simulink model "tank_reactor_no_error_dyn"  (R2020a)
settings: Solver=FixedStepAuto  StartTime=0.0  StopTime=options.T_train  FixedStep=options.dt  RelTol=1e-3
PreLoadFcn:
  | load PIDGainSchedExample.mat
model workspace (MAT data in the model file):
  op_snapshot1 : handle (value not decoded)
undefined symbols (not defined in the file or in its folder): C, Controllers, D, I, N, options, P, sigbuilder_block
libraries: neural x132, simulink x2, simulink_need_slupdate x1
(part 4 of 6)

== system tank_reactor_no_error_dyn/NN/Layer 3/Delays 1 ==
  "p{3}" : Inport  PortDimensions=30
      mask Display: e = 0.06;c1 = [120 230 180]/255;c2 = ([120 230 180]+0)/(256+128);c3 = ([120 230 180]+128)/(256+128);patch([0 1 1 0],[0 0 1 1],c1);patch([0 1 1 1-e 1-e 0+e],[0 0 1 1-e 0+e 0+e],c2);patch([0 0 1 1-e 0+e 0+e],[0 1 1 1-e 1-e 0+e],c3);plot([0 1 1 0 0],[0 0 1 1 0]);
  mux : Mux  Inputs=1
      mask Display: e = 0.06;c1 = [120 150 230]/255;c2 = ([120 150 230]+0)/383;c3 = ([120 150 230]+128)/383;patch([0 1 1 0],[0 0 1 1],c1);patch([0 1 1 1-e 1-e 0+e],[0 0 1 1-e 0+e 0+e],c2);patch([0 0 1 1-e 0+e 0+e],[0 1 1 1-e 1-e 0+e],c3);plot([0 1 1 0 0],[0 0 1 1 0]);disp('Mux')
  "pd{3,2}" : Outport
      mask Display: e = 0.06;c1 = [120 230 180]/255;c2 = ([120 230 180]+0)/(256+128);c3 = ([120 230 180]+128)/(256+128);patch([0 1 1 0],[0 0 1 1],c1);patch([0 1 1 1-e 1-e 0+e],[0 0 1 1-e 0+e 0+e],c2);patch([0 0 1 1-e 0+e 0+e],[0 1 1 1-e 1-e 0+e],c3);plot([0 1 1 0 0],[0 0 1 1 0]);
  wires:
  "p{3}"/1 -> mux/1
  mux/1 -> "pd{3,2}"/1

== system tank_reactor_no_error_dyn/NN/Layer 3/LW{3,2} ==
  "ad{3,2}" : Inport  PortDimensions=30
      mask Display: e = 0.06;c1 = [120 230 180]/255;c2 = ([120 230 180]+0)/(256+128);c3 = ([120 230 180]+128)/(256+128);patch([0 1 1 0],[0 0 1 1],c1);patch([0 1 1 1-e 1-e 0+e],[0 0 1 1-e 0+e 0+e],c2);patch([0 0 1 1-e 0+e 0+e],[0 1 1 1-e 1-e 0+e],c3);plot([0 1 1 0 0],[0 0 1 1 0]);
  "IW{3,2}(1,:)'" : Constant  Value=[-0.0511636272727241381286233945502317510545253753662109375;-0.228435345687879765019800970549113117158412933349609375;0.09378185793298553230012970516327186487615108489990234375;0.30732968004933403083356324714259244501590728759765625;-0.0026202039604571948812339332590681806323118507862091064453125;-0.1112622079165584698667856855536228977143764495849609375;-0.10130639427641263683455008504097349941730499267578125;0.06769739116965713121576442290461272932589054107666015625;-0.1255451148000425731776630300373653881251811981201171875;-0.07607780761738723585008159489007084630429744720458984375;-0.08226752934348340040582314713901723735034465789794921875;-0.01408145722205182519271016161610532435588538646697998046875;-0.02022664868012079286696547342216945253312587738037109375;-0.132883871763963157253130020762910135090351104736328125;-0.324757632621128611294381016705301590263843536376953125;-0.0153480898639730863053376452853626688010990619659423828125;0.01046282805957223123460853031474471208639442920684814453125;-0.00411317650747298861613199250086836400441825389862060546875;0.06722186949668589039941224427820998243987560272216796875;0.0896070865747360667530330147201311774551868438720703125;-0.254826262873892039895196148791001178324222564697265625;-0.02907748808419595432095405840300372801721096038818359375;0.1823688820218593298339015973397181369364261627197265625;-0.07852964486181500392003584920530556701123714447021484375;0.287449325203550654084239113217336125671863555908203125;-0.0266849151074926189963765210677593131549656391143798828125;0.041099048807482808920443773104125284589827060699462890625;0.081766120098062444743192145324428565800189971923828125;0.45293085224205065220104415857349522411823272705078125;-0.343650288483047849918960991999483667314052581787109375]
      mask Display: e = 0.06;c1 = [120 150 230]/255;c2 = ([120 150 230]+0)/383;c3 = ([120 150 230]+128)/383;patch([0 1 1 0],[0 0 1 1],c1);patch([0 1 1 1-e 1-e 0+e],[0 0 1 1-e 0+e 0+e],c2);patch([0 0 1 1-e 0+e 0+e],[0 1 1 1-e 1-e 0+e],c3);plot([0 1 1 0 0],[0 0 1 1 0]);disp('weights');
  Mux : Mux  Inputs=1
      mask Display: e = 0.06;c1 = [120 150 230]/255;c2 = ([120 150 230]+0)/383;c3 = ([120 150 230]+128)/383;patch([0 1 1 0],[0 0 1 1],c1);patch([0 1 1 1-e 1-e 0+e],[0 0 1 1-e 0+e 0+e],c2);patch([0 0 1 1-e 0+e 0+e],[0 1 1 1-e 1-e 0+e],c3);plot([0 1 1 0 0],[0 0 1 1 0]);disp('Mux');
  dotprod1 : neural/Weight Functions/dotprod
  "lz{3,2}" : Outport
      mask Display: e = 0.06;c1 = [120 230 180]/255;c2 = ([120 230 180]+0)/(256+128);c3 = ([120 230 180]+128)/(256+128);patch([0 1 1 0],[0 0 1 1],c1);patch([0 1 1 1-e 1-e 0+e],[0 0 1 1-e 0+e 0+e],c2);patch([0 0 1 1-e 0+e 0+e],[0 1 1 1-e 1-e 0+e],c3);plot([0 1 1 0 0],[0 0 1 1 0]);
  wires:
  "IW{3,2}(1,:)'"/1 -> dotprod1/1
  "ad{3,2}"/1 -> dotprod1/2
  dotprod1/1 -> Mux/1
  Mux/1 -> "lz{3,2}"/1

== system tank_reactor_no_error_dyn/NN_cex_1/Layer 1/Delays 1 ==
  "p{1}" : Inport  PortDimensions=8
      mask Display: e = 0.06;c1 = [120 230 180]/255;c2 = ([120 230 180]+0)/(256+128);c3 = ([120 230 180]+128)/(256+128);patch([0 1 1 0],[0 0 1 1],c1);patch([0 1 1 1-e 1-e 0+e],[0 0 1 1-e 0+e 0+e],c2);patch([0 0 1 1-e 0+e 0+e],[0 1 1 1-e 1-e 0+e],c3);plot([0 1 1 0 0],[0 0 1 1 0]);
  mux : Mux  Inputs=1
      mask Display: e = 0.06;c1 = [120 150 230]/255;c2 = ([120 150 230]+0)/383;c3 = ([120 150 230]+128)/383;patch([0 1 1 0],[0 0 1 1],c1);patch([0 1 1 1-e 1-e 0+e],[0 0 1 1-e 0+e 0+e],c2);patch([0 0 1 1-e 0+e 0+e],[0 1 1 1-e 1-e 0+e],c3);plot([0 1 1 0 0],[0 0 1 1 0]);disp('Mux')
  "pd{1,1}" : Outport
      mask Display: e = 0.06;c1 = [120 230 180]/255;c2 = ([120 230 180]+0)/(256+128);c3 = ([120 230 180]+128)/(256+128);patch([0 1 1 0],[0 0 1 1],c1);patch([0 1 1 1-e 1-e 0+e],[0 0 1 1-e 0+e 0+e],c2);patch([0 0 1 1-e 0+e 0+e],[0 1 1 1-e 1-e 0+e],c3);plot([0 1 1 0 0],[0 0 1 1 0]);
  wires:
  "p{1}"/1 -> mux/1
  mux/1 -> "pd{1,1}"/1

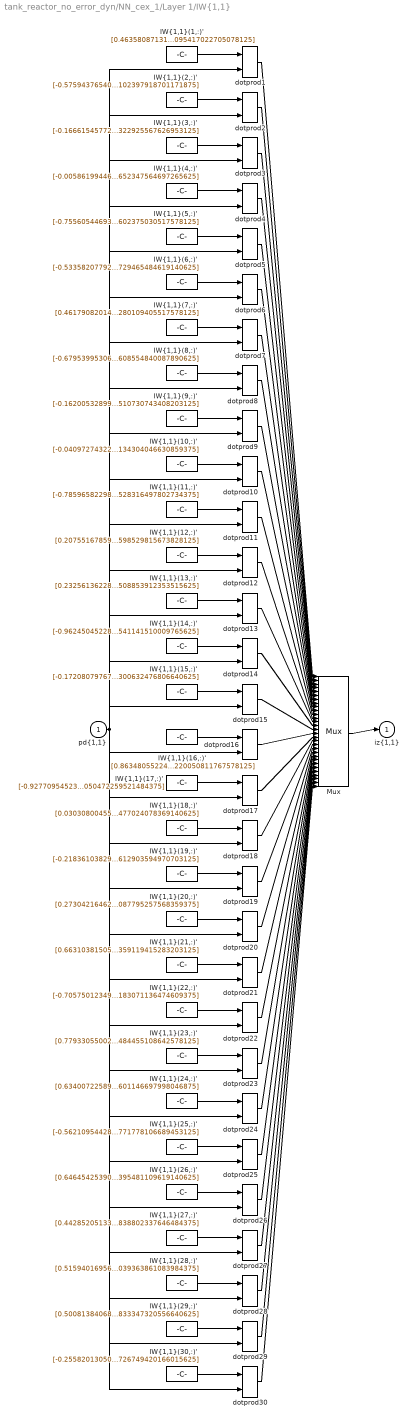
== system tank_reactor_no_error_dyn/NN_cex_1/Layer 1/IW{1,1} ==
  "pd{1,1}" : Inport  PortDimensions=8
      mask Display: e = 0.06;c1 = [120 230 180]/255;c2 = ([120 230 180]+0)/(256+128);c3 = ([120 230 180]+128)/(256+128);patch([0 1 1 0],[0 0 1 1],c1);patch([0 1 1 1-e 1-e 0+e],[0 0 1 1-e 0+e 0+e],c2);patch([0 0 1 1-e 0+e 0+e],[0 1 1 1-e 1-e 0+e],c3);plot([0 1 1 0 0],[0 0 1 1 0]);
  "IW{1,1}(1,:)'" : Constant  Value=[0.463580871318489851073962881855550222098827362060546875;-0.7904587112242886792756735303555615246295928955078125;0.57442801713559255016861015974427573382854461669921875;1.4978647593431768658689406947814859449863433837890625;-0.95724167897599621301907291126553900539875030517578125;0.064253678467424413245367986746714450418949127197265625;0.2444816783607909604913999146447167731821537017822265625;-0.2330448826646716320443175618493114598095417022705078125]
      mask Display: e = 0.06;c1 = [120 150 230]/255;c2 = ([120 150 230]+0)/383;c3 = ([120 150 230]+128)/383;patch([0 1 1 0],[0 0 1 1],c1);patch([0 1 1 1-e 1-e 0+e],[0 0 1 1-e 0+e 0+e],c2);patch([0 0 1 1-e 0+e 0+e],[0 1 1 1-e 1-e 0+e],c3);plot([0 1 1 0 0],[0 0 1 1 0]);disp('Weights');
  "IW{1,1}(10,:)'" : Constant  Value=[-0.040972743222529188489300366882162052206695079803466796875;1.3653833096036469552103653768426738679409027099609375;-0.91960544872284799566841684281826019287109375;-0.67287265316171274154299908332177437841892242431640625;-0.14617210117683787640174841726548038423061370849609375;0.380836409839925504883240137132816016674041748046875;0.0876222293789833683863577107331366278231143951416015625;1.256903587889906415142604600987397134304046630859375]
      mask Display: e = 0.06;c1 = [120 150 230]/255;c2 = ([120 150 230]+0)/383;c3 = ([120 150 230]+128)/383;patch([0 1 1 0],[0 0 1 1],c1);patch([0 1 1 1-e 1-e 0+e],[0 0 1 1-e 0+e 0+e],c2);patch([0 0 1 1-e 0+e 0+e],[0 1 1 1-e 1-e 0+e],c3);plot([0 1 1 0 0],[0 0 1 1 0]);disp('Weights');
  "IW{1,1}(11,:)'" : Constant  Value=[-0.7859658229803023754556079438771121203899383544921875;-0.52967905565982198456964624710963107645511627197265625;0.90365927008908764062056206967099569737911224365234375;-0.427517699502745929240887790001579560339450836181640625;-0.85982789438278517391012201187550090253353118896484375;-1.1238235294587177737213323780451901257038116455078125;-0.325401621469426693966653374445741064846515655517578125;-0.08553663223588357789051173085681512020528316497802734375]
      mask Display: e = 0.06;c1 = [120 150 230]/255;c2 = ([120 150 230]+0)/383;c3 = ([120 150 230]+128)/383;patch([0 1 1 0],[0 0 1 1],c1);patch([0 1 1 1-e 1-e 0+e],[0 0 1 1-e 0+e 0+e],c2);patch([0 0 1 1-e 0+e 0+e],[0 1 1 1-e 1-e 0+e],c3);plot([0 1 1 0 0],[0 0 1 1 0]);disp('Weights');
  "IW{1,1}(12,:)'" : Constant  Value=[0.2075516785995884794235877279788837768137454986572265625;-1.2880702182765999541658175076008774340152740478515625;0.55049483529810461224229811705299653112888336181640625;-0.3942878107891996108946841559372842311859130859375;0.78421997391049125258888352618669159710407257080078125;-0.0082326501651055657149402833283602376468479633331298828125;0.08183215105199100058985806072087143547832965850830078125;1.60118606217460968110799512942321598529815673828125]
      mask Display: e = 0.06;c1 = [120 150 230]/255;c2 = ([120 150 230]+0)/383;c3 = ([120 150 230]+128)/383;patch([0 1 1 0],[0 0 1 1],c1);patch([0 1 1 1-e 1-e 0+e],[0 0 1 1-e 0+e 0+e],c2);patch([0 0 1 1-e 0+e 0+e],[0 1 1 1-e 1-e 0+e],c3);plot([0 1 1 0 0],[0 0 1 1 0]);disp('Weights');
  "IW{1,1}(13,:)'" : Constant  Value=[0.2325613622819835690780365666796569712460041046142578125;0.6884494995406864603637586697004735469818115234375;0.91152589192887567559608896772260777652263641357421875;-0.974281841732740350181529720430262386798858642578125;0.561050562518456530369803658686578273773193359375;-0.36138030563152911955882018446573056280612945556640625;0.031805128071507038356457996997050940990447998046875;1.3856379731621599749047391014755703508853912353515625]
      mask Display: e = 0.06;c1 = [120 150 230]/255;c2 = ([120 150 230]+0)/383;c3 = ([120 150 230]+128)/383;patch([0 1 1 0],[0 0 1 1],c1);patch([0 1 1 1-e 1-e 0+e],[0 0 1 1-e 0+e 0+e],c2);patch([0 0 1 1-e 0+e 0+e],[0 1 1 1-e 1-e 0+e],c3);plot([0 1 1 0 0],[0 0 1 1 0]);disp('Weights');
  "IW{1,1}(14,:)'" : Constant  Value=[-0.96245045228366199463465591179556213319301605224609375;-1.2333069155908173986091469487291760742664337158203125;0.79278077813697100939549500253633596003055572509765625;0.6794397573296786507768274532281793653964996337890625;-0.527000734411264826206888756132684648036956787109375;0.787959872679240280746171265491284430027008056640625;-0.61877659409885932273454045571270398795604705810546875;-0.74362758890356295271573117133812047541141510009765625]
      mask Display: e = 0.06;c1 = [120 150 230]/255;c2 = ([120 150 230]+0)/383;c3 = ([120 150 230]+128)/383;patch([0 1 1 0],[0 0 1 1],c1);patch([0 1 1 1-e 1-e 0+e],[0 0 1 1-e 0+e 0+e],c2);patch([0 0 1 1-e 0+e 0+e],[0 1 1 1-e 1-e 0+e],c3);plot([0 1 1 0 0],[0 0 1 1 0]);disp('Weights');
  "IW{1,1}(15,:)'" : Constant  Value=[-0.1720807976720290788374967405616189353168010711669921875;1.6346800282565066009254906020942144095897674560546875;-1.5275045226209156279395529054454527795314788818359375;0.48163706898306113401986294775269925594329833984375;-1.4090195244134176011385761739802546799182891845703125;1.0074444406116940253781422143219970166683197021484375;0.149048248710748676426618430923554114997386932373046875;0.583897769695257640165664270170964300632476806640625]
      mask Display: e = 0.06;c1 = [120 150 230]/255;c2 = ([120 150 230]+0)/383;c3 = ([120 150 230]+128)/383;patch([0 1 1 0],[0 0 1 1],c1);patch([0 1 1 1-e 1-e 0+e],[0 0 1 1-e 0+e 0+e],c2);patch([0 0 1 1-e 0+e 0+e],[0 1 1 1-e 1-e 0+e],c3);plot([0 1 1 0 0],[0 0 1 1 0]);disp('Weights');
  "IW{1,1}(16,:)'" : Constant  Value=[0.8634805522466171279205582322902046144008636474609375;-0.826832306692147245286150791798718273639678955078125;-0.459024428825649588592483496540808118879795074462890625;-0.225724673917949036905383763951249420642852783203125;0.7769046624413535884201564840623177587985992431640625;0.07897558014084467281623602730178390629589557647705078125;-0.80444668751484471602708481441368348896503448486328125;-0.68029164592008506406983769920771010220050811767578125]
      mask Display: e = 0.06;c1 = [120 150 230]/255;c2 = ([120 150 230]+0)/383;c3 = ([120 150 230]+128)/383;patch([0 1 1 0],[0 0 1 1],c1);patch([0 1 1 1-e 1-e 0+e],[0 0 1 1-e 0+e 0+e],c2);patch([0 0 1 1-e 0+e 0+e],[0 1 1 1-e 1-e 0+e],c3);plot([0 1 1 0 0],[0 0 1 1 0]);disp('Weights');
  "IW{1,1}(17,:)'" : Constant  Value=[-0.92770954523786175460742242648848332464694976806640625;-0.70379974998822880660753753545577637851238250732421875;0.49312602053411913605174277108744718134403228759765625;0.2053519305894300484016667951436829753220081329345703125;0.81354542032451415689564555577817372977733612060546875;0.06332053666104490996513476375184836797416210174560546875;0.392478721046141398876017092334222979843616485595703125;0.9425610515299085445661830817698501050472259521484375]
      mask Display: e = 0.06;c1 = [120 150 230]/255;c2 = ([120 150 230]+0)/383;c3 = ([120 150 230]+128)/383;patch([0 1 1 0],[0 0 1 1],c1);patch([0 1 1 1-e 1-e 0+e],[0 0 1 1-e 0+e 0+e],c2);patch([0 0 1 1-e 0+e 0+e],[0 1 1 1-e 1-e 0+e],c3);plot([0 1 1 0 0],[0 0 1 1 0]);disp('Weights');
  "IW{1,1}(18,:)'" : Constant  Value=[0.030308004556539668017389743681633262895047664642333984375;0.72396828867836060528162533955764956772327423095703125;0.59124165685490748245456416043452918529510498046875;0.68453876641339650443995878958958201110363006591796875;0.873486939293690145547088832245208323001861572265625;-0.55859954329883254597888253556448034942150115966796875;0.88615609615319101965980053137172944843769073486328125;0.8792828693653904625904260683455504477024078369140625]
      mask Display: e = 0.06;c1 = [120 150 230]/255;c2 = ([120 150 230]+0)/383;c3 = ([120 150 230]+128)/383;patch([0 1 1 0],[0 0 1 1],c1);patch([0 1 1 1-e 1-e 0+e],[0 0 1 1-e 0+e 0+e],c2);patch([0 0 1 1-e 0+e 0+e],[0 1 1 1-e 1-e 0+e],c3);plot([0 1 1 0 0],[0 0 1 1 0]);disp('Weights');
  "IW{1,1}(19,:)'" : Constant  Value=[-0.21836103829253905583840378312743268907070159912109375;-1.7653401894298923480164376087486743927001953125;0.1304230755661318907900891872486681677401065826416015625;0.491037568941755153684169954431126825511455535888671875;0.880852994496023722348354567657224833965301513671875;0.4235760813815658831771315817604772746562957763671875;0.66282600456369278330015504252514801919460296630859375;-0.9759379388789650722202395627391524612903594970703125]
      mask Display: e = 0.06;c1 = [120 150 230]/255;c2 = ([120 150 230]+0)/383;c3 = ([120 150 230]+128)/383;patch([0 1 1 0],[0 0 1 1],c1);patch([0 1 1 1-e 1-e 0+e],[0 0 1 1-e 0+e 0+e],c2);patch([0 0 1 1-e 0+e 0+e],[0 1 1 1-e 1-e 0+e],c3);plot([0 1 1 0 0],[0 0 1 1 0]);disp('Weights');
  "IW{1,1}(2,:)'" : Constant  Value=[-0.57594376540703728917236503548338077962398529052734375;0.3962711625510093593760529984137974679470062255859375;-0.136957085468368655600812644479447044432163238525390625;0.90856087701288401614618805979262106120586395263671875;0.79920507598837442486683357856236398220062255859375;0.34068887162910421739780986172263510525226593017578125;0.94500832838045678574445673802983947098255157470703125;0.898124703405627666796817720751278102397918701171875]
      mask Display: e = 0.06;c1 = [120 150 230]/255;c2 = ([120 150 230]+0)/383;c3 = ([120 150 230]+128)/383;patch([0 1 1 0],[0 0 1 1],c1);patch([0 1 1 1-e 1-e 0+e],[0 0 1 1-e 0+e 0+e],c2);patch([0 0 1 1-e 0+e 0+e],[0 1 1 1-e 1-e 0+e],c3);plot([0 1 1 0 0],[0 0 1 1 0]);disp('Weights');
  "IW{1,1}(20,:)'" : Constant  Value=[0.27304216462729680170440360598149709403514862060546875;-1.2509692414445792163490978055051527917385101318359375;-0.59360848828293211187911992965382523834705352783203125;0.368084973461381192993968625160050578415393829345703125;-0.69093934225117104030999826136394403874874114990234375;0.52517178272850462139587079946068115532398223876953125;0.404032973990806620889770783833228051662445068359375;1.331038799733446520434654303244315087795257568359375]
      mask Display: e = 0.06;c1 = [120 150 230]/255;c2 = ([120 150 230]+0)/383;c3 = ([120 150 230]+128)/383;patch([0 1 1 0],[0 0 1 1],c1);patch([0 1 1 1-e 1-e 0+e],[0 0 1 1-e 0+e 0+e],c2);patch([0 0 1 1-e 0+e 0+e],[0 1 1 1-e 1-e 0+e],c3);plot([0 1 1 0 0],[0 0 1 1 0]);disp('Weights');
  "IW{1,1}(21,:)'" : Constant  Value=[0.66310381505613558150713515715324319899082183837890625;-0.5068485717960167225015766234719194471836090087890625;0.12251030924586096826356396150004002265632152557373046875;-0.453308562938941894682187694343156181275844573974609375;-1.4355076890545730439185945215285755693912506103515625;0.3534278437696298791337312650284729897975921630859375;-0.5361448701653539483658050812664441764354705810546875;-1.144453668082821451434938353486359119415283203125]
      mask Display: e = 0.06;c1 = [120 150 230]/255;c2 = ([120 150 230]+0)/383;c3 = ([120 150 230]+128)/383;patch([0 1 1 0],[0 0 1 1],c1);patch([0 1 1 1-e 1-e 0+e],[0 0 1 1-e 0+e 0+e],c2);patch([0 0 1 1-e 0+e 0+e],[0 1 1 1-e 1-e 0+e],c3);plot([0 1 1 0 0],[0 0 1 1 0]);disp('Weights');
  "IW{1,1}(22,:)'" : Constant  Value=[-0.7057501234978935666930510706151835620403289794921875;1.0777498783723895581232454787823371589183807373046875;0.9181709250255909449123237209278158843517303466796875;0.562010005880240637310407691984437406063079833984375;0.19714460918516607534911599941551685333251953125;1.147996642267212319410418785992078483104705810546875;-0.379426862334607761795268743298947811126708984375;-0.2291945269754227521019629421061836183071136474609375]
      mask Display: e = 0.06;c1 = [120 150 230]/255;c2 = ([120 150 230]+0)/383;c3 = ([120 150 230]+128)/383;patch([0 1 1 0],[0 0 1 1],c1);patch([0 1 1 1-e 1-e 0+e],[0 0 1 1-e 0+e 0+e],c2);patch([0 0 1 1-e 0+e 0+e],[0 1 1 1-e 1-e 0+e],c3);plot([0 1 1 0 0],[0 0 1 1 0]);disp('Weights');
  "IW{1,1}(23,:)'" : Constant  Value=[0.7793305500246863193325452812132425606250762939453125;-1.3963545070225931166163491070619784295558929443359375;-0.0197291050812327221908315522114207851700484752655029296875;0.6738974988460924020472475604037754237651824951171875;0.518831908117893814136323271668516099452972412109375;0.2877058771797831315808480212581343948841094970703125;-0.338558398751864164655245303947594948112964630126953125;-1.0022153826101807272408450444345362484455108642578125]
      mask Display: e = 0.06;c1 = [120 150 230]/255;c2 = ([120 150 230]+0)/383;c3 = ([120 150 230]+128)/383;patch([0 1 1 0],[0 0 1 1],c1);patch([0 1 1 1-e 1-e 0+e],[0 0 1 1-e 0+e 0+e],c2);patch([0 0 1 1-e 0+e 0+e],[0 1 1 1-e 1-e 0+e],c3);plot([0 1 1 0 0],[0 0 1 1 0]);disp('Weights');
  "IW{1,1}(24,:)'" : Constant  Value=[0.6340072258966429341597859092871658504009246826171875;0.37790605979201341568796124192886054515838623046875;-0.85645656739814957081335933253285475075244903564453125;-0.307011093371232057780417790127103216946125030517578125;0.3271156209610583953661944178747944533824920654296875;-0.05214857299869594953189988473241101019084453582763671875;1.3630762535353053710451831648242659866809844970703125;-1.1632957683929685543944287928752601146697998046875]
      mask Display: e = 0.06;c1 = [120 150 230]/255;c2 = ([120 150 230]+0)/383;c3 = ([120 150 230]+128)/383;patch([0 1 1 0],[0 0 1 1],c1);patch([0 1 1 1-e 1-e 0+e],[0 0 1 1-e 0+e 0+e],c2);patch([0 0 1 1-e 0+e 0+e],[0 1 1 1-e 1-e 0+e],c3);plot([0 1 1 0 0],[0 0 1 1 0]);disp('Weights');
  "IW{1,1}(25,:)'" : Constant  Value=[-0.56210954428920822945059398989542387425899505615234375;-0.36545828277500336245253720335313118994235992431640625;1.0061415530919173288992851666989736258983612060546875;-0.75339005875760989283662638626992702484130859375;0.80492991378725620155165643154759891331195831298828125;-0.01355985355531138907003718685473359073512256145477294921875;-0.449973166387047929237752441622433252632617950439453125;1.13479554730583931387855045613832771778106689453125]
      mask Display: e = 0.06;c1 = [120 150 230]/255;c2 = ([120 150 230]+0)/383;c3 = ([120 150 230]+128)/383;patch([0 1 1 0],[0 0 1 1],c1);patch([0 1 1 1-e 1-e 0+e],[0 0 1 1-e 0+e 0+e],c2);patch([0 0 1 1-e 0+e 0+e],[0 1 1 1-e 1-e 0+e],c3);plot([0 1 1 0 0],[0 0 1 1 0]);disp('Weights');
  "IW{1,1}(26,:)'" : Constant  Value=[0.64645425390136879162383820585091598331928253173828125;0.5379115281036155327143433169112540781497955322265625;0.98482449266796734388407230653683654963970184326171875;-1.234152891743236946098249973147176206111907958984375;0.552845338795752372362812820938415825366973876953125;-0.74973727573836124182804496740573085844516754150390625;-0.39753604357000338342942313829553313553333282470703125;0.37774497687728614270241678241291083395481109619140625]
      mask Display: e = 0.06;c1 = [120 150 230]/255;c2 = ([120 150 230]+0)/383;c3 = ([120 150 230]+128)/383;patch([0 1 1 0],[0 0 1 1],c1);patch([0 1 1 1-e 1-e 0+e],[0 0 1 1-e 0+e 0+e],c2);patch([0 0 1 1-e 0+e 0+e],[0 1 1 1-e 1-e 0+e],c3);plot([0 1 1 0 0],[0 0 1 1 0]);disp('Weights');
  "IW{1,1}(27,:)'" : Constant  Value=[0.442852051339611085811753810048685409128665924072265625;-0.1612759616178441046674407743921619839966297149658203125;-1.059514801227666946914496293175034224987030029296875;-0.31801079923491604173335645100451074540615081787109375;1.31667604694982731672325826366432011127471923828125;-0.196637959511739401907703950200811959803104400634765625;-0.84257433986396723657463780909893102943897247314453125;-0.73562573460771873978814028305350802838802337646484375]
      mask Display: e = 0.06;c1 = [120 150 230]/255;c2 = ([120 150 230]+0)/383;c3 = ([120 150 230]+128)/383;patch([0 1 1 0],[0 0 1 1],c1);patch([0 1 1 1-e 1-e 0+e],[0 0 1 1-e 0+e 0+e],c2);patch([0 0 1 1-e 0+e 0+e],[0 1 1 1-e 1-e 0+e],c3);plot([0 1 1 0 0],[0 0 1 1 0]);disp('Weights');
  "IW{1,1}(28,:)'" : Constant  Value=[0.515940169569911066815848244004882872104644775390625;0.326390302099289819626193320800666697323322296142578125;0.79363286471308303049454480060376226902008056640625;0.53611866584574408012286994562600739300251007080078125;-0.87791311431382024199621127991122193634510040283203125;-0.1311120155577295831594852870694012381136417388916015625;1.1060321036358544688482652418315410614013671875;-0.81245786194538227587003120788722299039363861083984375]
      mask Display: e = 0.06;c1 = [120 150 230]/255;c2 = ([120 150 230]+0)/383;c3 = ([120 150 230]+128)/383;patch([0 1 1 0],[0 0 1 1],c1);patch([0 1 1 1-e 1-e 0+e],[0 0 1 1-e 0+e 0+e],c2);patch([0 0 1 1-e 0+e 0+e],[0 1 1 1-e 1-e 0+e],c3);plot([0 1 1 0 0],[0 0 1 1 0]);disp('Weights');
  "IW{1,1}(29,:)'" : Constant  Value=[0.50081384068591983105278586663189344108104705810546875;0.70784116501752458727736438959254883229732513427734375;-0.54083562909659033124398774816654622554779052734375;-0.4016607451257583338843915043980814516544342041015625;-0.637187205003586942808624371537007391452789306640625;-1.3621243366178481526418408975587226450443267822265625;1.1372953341399416604673433539574034512042999267578125;-0.7814124788651357622626392185338772833347320556640625]
      mask Display: e = 0.06;c1 = [120 150 230]/255;c2 = ([120 150 230]+0)/383;c3 = ([120 150 230]+128)/383;patch([0 1 1 0],[0 0 1 1],c1);patch([0 1 1 1-e 1-e 0+e],[0 0 1 1-e 0+e 0+e],c2);patch([0 0 1 1-e 0+e 0+e],[0 1 1 1-e 1-e 0+e],c3);plot([0 1 1 0 0],[0 0 1 1 0]);disp('Weights');
  "IW{1,1}(3,:)'" : Constant  Value=[-0.1666154577238947442907601725892163813114166259765625;-0.6536488119383376815818564864457584917545318603515625;-1.0562606311580997608956522526568733155727386474609375;1.135074772634802275916854341630823910236358642578125;0.631701996163486878543835700838826596736907958984375;-1.0490198465701379149095373577438294887542724609375;-0.281305602571892687802090904369833879172801971435546875;-0.2419406811468441109713722880769637413322925567626953125]
      mask Display: e = 0.06;c1 = [120 150 230]/255;c2 = ([120 150 230]+0)/383;c3 = ([120 150 230]+128)/383;patch([0 1 1 0],[0 0 1 1],c1);patch([0 1 1 1-e 1-e 0+e],[0 0 1 1-e 0+e 0+e],c2);patch([0 0 1 1-e 0+e 0+e],[0 1 1 1-e 1-e 0+e],c3);plot([0 1 1 0 0],[0 0 1 1 0]);disp('Weights');
  "IW{1,1}(30,:)'" : Constant  Value=[-0.255820130507038723255419654378783889114856719970703125;-0.42046638486646104038158000548719428479671478271484375;0.94480030775071865978276264286250807344913482666015625;1.46246777067761968282866291701793670654296875;-0.94321670011016112145085799056687392294406890869140625;-0.131027866533403980486838236174662597477436065673828125;0.97966607272397465688840156872174702584743499755859375;-0.414381316283911671494166739648790098726749420166015625]
      mask Display: e = 0.06;c1 = [120 150 230]/255;c2 = ([120 150 230]+0)/383;c3 = ([120 150 230]+128)/383;patch([0 1 1 0],[0 0 1 1],c1);patch([0 1 1 1-e 1-e 0+e],[0 0 1 1-e 0+e 0+e],c2);patch([0 0 1 1-e 0+e 0+e],[0 1 1 1-e 1-e 0+e],c3);plot([0 1 1 0 0],[0 0 1 1 0]);disp('Weights');
  "IW{1,1}(4,:)'" : Constant  Value=[-0.005861994462960277464669278657538598054088652133941650390625;0.310384610035220942503286778446636162698268890380859375;-0.303985715566599645764966908245696686208248138427734375;1.532457273094987026951230291160754859447479248046875;0.14221060335721869005709550037863664329051971435546875;-0.2424428009628119828899883714257157407701015472412109375;0.78518710237456657008436877731583081185817718505859375;1.1900275375553894807723054327652789652347564697265625]
      mask Display: e = 0.06;c1 = [120 150 230]/255;c2 = ([120 150 230]+0)/383;c3 = ([120 150 230]+128)/383;patch([0 1 1 0],[0 0 1 1],c1);patch([0 1 1 1-e 1-e 0+e],[0 0 1 1-e 0+e 0+e],c2);patch([0 0 1 1-e 0+e 0+e],[0 1 1 1-e 1-e 0+e],c3);plot([0 1 1 0 0],[0 0 1 1 0]);disp('Weights');
  "IW{1,1}(5,:)'" : Constant  Value=[-0.7556054469320427902090386851341463625431060791015625;-1.1675269259961778001155607853434048593044281005859375;0.357343037332967627950353062260546721518039703369140625;-1.2615101675971087669125836328021250665187835693359375;0.318800595041070999879906366913928650319576263427734375;0.11144197081600955290259236107885953970253467559814453125;0.331933459356202720247352999649592675268650054931640625;0.1749402223806457989940810193729703314602375030517578125]
      mask Display: e = 0.06;c1 = [120 150 230]/255;c2 = ([120 150 230]+0)/383;c3 = ([120 150 230]+128)/383;patch([0 1 1 0],[0 0 1 1],c1);patch([0 1 1 1-e 1-e 0+e],[0 0 1 1-e 0+e 0+e],c2);patch([0 0 1 1-e 0+e 0+e],[0 1 1 1-e 1-e 0+e],c3);plot([0 1 1 0 0],[0 0 1 1 0]);disp('Weights');
  "IW{1,1}(6,:)'" : Constant  Value=[-0.533582077924919406797243937035091221332550048828125;-0.1769956811210130764866477193208993412554264068603515625;-0.68676284949857790973481996843474917113780975341796875;-0.2768405634972224138579122154624201357364654541015625;-0.85842097286933805033726230249158106744289398193359375;0.317723199909580367172878823112114332616329193115234375;-1.10436479719843827496106314356438815593719482421875;0.8243658839545775496304713669815100729465484619140625]
      mask Display: e = 0.06;c1 = [120 150 230]/255;c2 = ([120 150 230]+0)/383;c3 = ([120 150 230]+128)/383;patch([0 1 1 0],[0 0 1 1],c1);patch([0 1 1 1-e 1-e 0+e],[0 0 1 1-e 0+e 0+e],c2);patch([0 0 1 1-e 0+e 0+e],[0 1 1 1-e 1-e 0+e],c3);plot([0 1 1 0 0],[0 0 1 1 0]);disp('Weights');
  "IW{1,1}(7,:)'" : Constant  Value=[0.461790820143882341231034160955459810793399810791015625;0.9523723514546293955618239124305546283721923828125;-0.86591776759901872839719771945965476334095001220703125;0.2034614325072331142418846638975082896649837493896484375;-1.0535322448098103365055067115463316440582275390625;0.96893238416265947687833204327034763991832733154296875;0.5560285087582921281779135824763216078281402587890625;-0.73762414930330699736060751092736609280109405517578125]
      mask Display: e = 0.06;c1 = [120 150 230]/255;c2 = ([120 150 230]+0)/383;c3 = ([120 150 230]+128)/383;patch([0 1 1 0],[0 0 1 1],c1);patch([0 1 1 1-e 1-e 0+e],[0 0 1 1-e 0+e 0+e],c2);patch([0 0 1 1-e 0+e 0+e],[0 1 1 1-e 1-e 0+e],c3);plot([0 1 1 0 0],[0 0 1 1 0]);disp('Weights');
  "IW{1,1}(8,:)'" : Constant  Value=[-0.679539953065417368094358607777394354343414306640625;-0.675914190639570033880545452120713889598846435546875;-0.97077223646583943317267539896420203149318695068359375;-0.08346642929951418599099355333237326703965663909912109375;-0.98150656874792618911129693515249527990818023681640625;0.732775463199345278297869299422018229961395263671875;0.89468062331483999560788333837990649044513702392578125;-0.57336653345065580200667909593903459608554840087890625]
      mask Display: e = 0.06;c1 = [120 150 230]/255;c2 = ([120 150 230]+0)/383;c3 = ([120 150 230]+128)/383;patch([0 1 1 0],[0 0 1 1],c1);patch([0 1 1 1-e 1-e 0+e],[0 0 1 1-e 0+e 0+e],c2);patch([0 0 1 1-e 0+e 0+e],[0 1 1 1-e 1-e 0+e],c3);plot([0 1 1 0 0],[0 0 1 1 0]);disp('Weights');
  "IW{1,1}(9,:)'" : Constant  Value=[-0.162005328993866937192791510824463330209255218505859375;0.6545225265598786368315131767303682863712310791015625;0.0250481552224244528870311654600300244055688381195068359375;-0.0685849802281766340872337650580448098480701446533203125;-1.366024248471656932224504998885095119476318359375;0.8217145446568496769401690471568144857883453369140625;-1.1737162817449757756804729069699533283710479736328125;0.0134397026919535929334603707729911548085510730743408203125]
      mask Display: e = 0.06;c1 = [120 150 230]/255;c2 = ([120 150 230]+0)/383;c3 = ([120 150 230]+128)/383;patch([0 1 1 0],[0 0 1 1],c1);patch([0 1 1 1-e 1-e 0+e],[0 0 1 1-e 0+e 0+e],c2);patch([0 0 1 1-e 0+e 0+e],[0 1 1 1-e 1-e 0+e],c3);plot([0 1 1 0 0],[0 0 1 1 0]);disp('Weights');
  Mux : Mux  Inputs=30
      mask Display: e = 0.06;c1 = [120 150 230]/255;c2 = ([120 150 230]+0)/383;c3 = ([120 150 230]+128)/383;patch([0 1 1 0],[0 0 1 1],c1);patch([0 1 1 1-e 1-e 0+e],[0 0 1 1-e 0+e 0+e],c2);patch([0 0 1 1-e 0+e 0+e],[0 1 1 1-e 1-e 0+e],c3);plot([0 1 1 0 0],[0 0 1 1 0]);disp('Mux');
  dotprod{1..30} (30 alike) : neural/Weight Functions/dotprod
  "iz{1,1}" : Outport
      mask Display: e = 0.06;c1 = [120 230 180]/255;c2 = ([120 230 180]+0)/(256+128);c3 = ([120 230 180]+128)/(256+128);patch([0 1 1 0],[0 0 1 1],c1);patch([0 1 1 1-e 1-e 0+e],[0 0 1 1-e 0+e 0+e],c2);patch([0 0 1 1-e 0+e 0+e],[0 1 1 1-e 1-e 0+e],c3);plot([0 1 1 0 0],[0 0 1 1 0]);
  wires:
  "IW{1,1}(1,:)'"/1 -> dotprod1/1
  "pd{1,1}"/1 -> dotprod1/2, dotprod2/2, dotprod3/2, dotprod4/2, dotprod5/2, dotprod6/2, dotprod7/2, dotprod8/2, dotprod9/2, dotprod10/2, dotprod11/2, dotprod12/2, dotprod13/2, dotprod14/2, dotprod15/2, dotprod16/2, dotprod17/2, dotprod18/2, dotprod19/2, dotprod20/2, dotprod21/2, dotprod22/2, dotprod23/2, dotprod24/2, dotprod25/2, dotprod26/2, dotprod27/2, dotprod28/2, dotprod29/2, dotprod30/2
  dotprod1/1 -> Mux/1
  "IW{1,1}(2,:)'"/1 -> dotprod2/1
  dotprod2/1 -> Mux/2
  "IW{1,1}(3,:)'"/1 -> dotprod3/1
  dotprod3/1 -> Mux/3
  "IW{1,1}(4,:)'"/1 -> dotprod4/1
  dotprod4/1 -> Mux/4
  "IW{1,1}(5,:)'"/1 -> dotprod5/1
  dotprod5/1 -> Mux/5
  "IW{1,1}(6,:)'"/1 -> dotprod6/1
  dotprod6/1 -> Mux/6
  "IW{1,1}(7,:)'"/1 -> dotprod7/1
  dotprod7/1 -> Mux/7
  "IW{1,1}(8,:)'"/1 -> dotprod8/1
  dotprod8/1 -> Mux/8
  "IW{1,1}(9,:)'"/1 -> dotprod9/1
  dotprod9/1 -> Mux/9
  "IW{1,1}(10,:)'"/1 -> dotprod10/1
  dotprod10/1 -> Mux/10
  "IW{1,1}(11,:)'"/1 -> dotprod11/1
  dotprod11/1 -> Mux/11
  "IW{1,1}(12,:)'"/1 -> dotprod12/1
  dotprod12/1 -> Mux/12
  "IW{1,1}(13,:)'"/1 -> dotprod13/1
  dotprod13/1 -> Mux/13
  "IW{1,1}(14,:)'"/1 -> dotprod14/1
  dotprod14/1 -> Mux/14
  "IW{1,1}(15,:)'"/1 -> dotprod15/1
  dotprod15/1 -> Mux/15
  "IW{1,1}(16,:)'"/1 -> dotprod16/1
  dotprod16/1 -> Mux/16
  "IW{1,1}(17,:)'"/1 -> dotprod17/1
  dotprod17/1 -> Mux/17
  "IW{1,1}(18,:)'"/1 -> dotprod18/1
  dotprod18/1 -> Mux/18
  "IW{1,1}(19,:)'"/1 -> dotprod19/1
  dotprod19/1 -> Mux/19
  "IW{1,1}(20,:)'"/1 -> dotprod20/1
  dotprod20/1 -> Mux/20
  "IW{1,1}(21,:)'"/1 -> dotprod21/1
  dotprod21/1 -> Mux/21
  "IW{1,1}(22,:)'"/1 -> dotprod22/1
  dotprod22/1 -> Mux/22
  "IW{1,1}(23,:)'"/1 -> dotprod23/1
  dotprod23/1 -> Mux/23
  "IW{1,1}(24,:)'"/1 -> dotprod24/1
  dotprod24/1 -> Mux/24
  "IW{1,1}(25,:)'"/1 -> dotprod25/1
  dotprod25/1 -> Mux/25
  "IW{1,1}(26,:)'"/1 -> dotprod26/1
  dotprod26/1 -> Mux/26
  "IW{1,1}(27,:)'"/1 -> dotprod27/1
  dotprod27/1 -> Mux/27
  "IW{1,1}(28,:)'"/1 -> dotprod28/1
  dotprod28/1 -> Mux/28
  "IW{1,1}(29,:)'"/1 -> dotprod29/1
  dotprod29/1 -> Mux/29
  "IW{1,1}(30,:)'"/1 -> dotprod30/1
  dotprod30/1 -> Mux/30
  Mux/1 -> "iz{1,1}"/1

== system tank_reactor_no_error_dyn/NN_cex_1/Layer 2/Delays 1 ==
  "p{2}" : Inport  PortDimensions=30
      mask Display: e = 0.06;c1 = [120 230 180]/255;c2 = ([120 230 180]+0)/(256+128);c3 = ([120 230 180]+128)/(256+128);patch([0 1 1 0],[0 0 1 1],c1);patch([0 1 1 1-e 1-e 0+e],[0 0 1 1-e 0+e 0+e],c2);patch([0 0 1 1-e 0+e 0+e],[0 1 1 1-e 1-e 0+e],c3);plot([0 1 1 0 0],[0 0 1 1 0]);
  mux : Mux  Inputs=1
      mask Display: e = 0.06;c1 = [120 150 230]/255;c2 = ([120 150 230]+0)/383;c3 = ([120 150 230]+128)/383;patch([0 1 1 0],[0 0 1 1],c1);patch([0 1 1 1-e 1-e 0+e],[0 0 1 1-e 0+e 0+e],c2);patch([0 0 1 1-e 0+e 0+e],[0 1 1 1-e 1-e 0+e],c3);plot([0 1 1 0 0],[0 0 1 1 0]);disp('Mux')
  "pd{2,1}" : Outport
      mask Display: e = 0.06;c1 = [120 230 180]/255;c2 = ([120 230 180]+0)/(256+128);c3 = ([120 230 180]+128)/(256+128);patch([0 1 1 0],[0 0 1 1],c1);patch([0 1 1 1-e 1-e 0+e],[0 0 1 1-e 0+e 0+e],c2);patch([0 0 1 1-e 0+e 0+e],[0 1 1 1-e 1-e 0+e],c3);plot([0 1 1 0 0],[0 0 1 1 0]);
  wires:
  "p{2}"/1 -> mux/1
  mux/1 -> "pd{2,1}"/1
